simulink model "tipologia_2_valutazioni_extra"  (R2022a)
settings: Solver=VariableStepAuto  StartTime=0.0  StopTime=10.0  RelTol=1e-3
values from neighbouring files (symbols this model uses):
  K_r = 1    [tipologia_2.m]
libraries: cstblocks x3
settings Model: Creator=giuli  LastModifiedBy=giuli

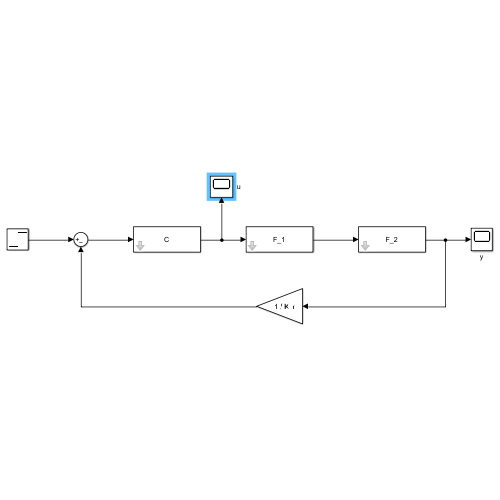
[thumbnail: Simulink's stored preview of the top-level diagram]
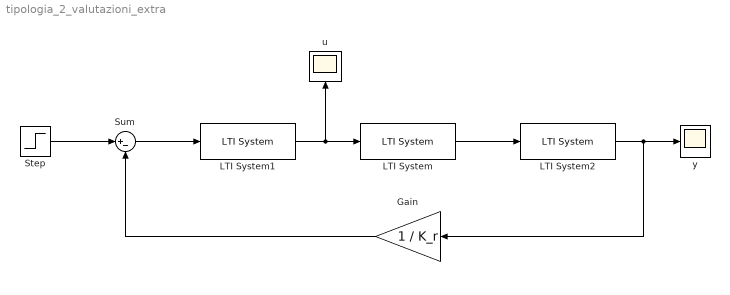
== system tipologia_2_valutazioni_extra ==
  Gain : Gain  Gain=1 / K_r
  LTI System : cstblocks/LTI System  sys=F_1  IC=[]
  LTI System1 : cstblocks/LTI System  sys=C  IC=[]
  LTI System2 : cstblocks/LTI System  sys=F_2  IC=[]
  Step : Step  SampleTime=0
  Sum : Sum  Inputs=|+-
  u : Scope
  y : Scope
  wires:
  LTI System1/1 -> u/1, LTI System/1
  LTI System/1 -> LTI System2/1
  Step/1 -> Sum/1
  Sum/1 -> LTI System1/1
  Gain/1 -> Sum/2
  LTI System2/1 -> Gain/1, y/1
